simulink model "spectrum_analyzer"  (R2017a)
settings: Solver=VariableStepDiscrete  StartTime=0.0  StopTime=10.0  MaxStep=0.03  RelTol=1e-3
settings Model: Creator=Naveed  LastModifiedBy=Naveed

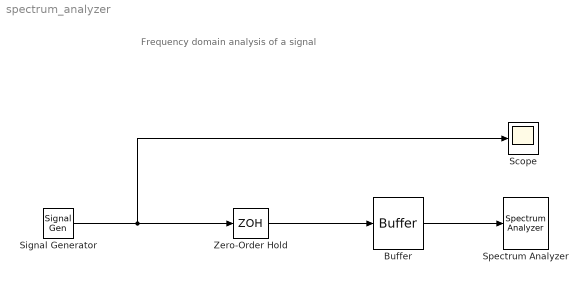
== system spectrum_analyzer ==
  note: Frequency domain analysis of a signal
  Buffer : Buffer  N=512  OutputFrames=off
  Scope : Scope
  Signal Generator : SignalGenerator  WaveForm=sawtooth  Amplitude=5  Frequency=5
  Spectrum Analyzer : SpectrumAnalyzer
  Zero-Order Hold : ZeroOrderHold  SampleTime=0.001
  wires:
  Signal Generator/1 -> Scope/1, Zero-Order Hold/1
  Zero-Order Hold/1 -> Buffer/1
  Buffer/1 -> Spectrum Analyzer/1
